simulink model "test_ntc"  (R2018a)
settings: Solver=ode1  StartTime=0.0  StopTime=8  FixedStep=1e-3  RelTol=1e-3
undefined symbols (not defined in the file): ntc10k
libraries: fl_lib x19, nesl_utility x6, elec_lib x2, simulink x2
settings Model: Creator=ChLan  LastModifiedBy=ChLan
settings SimscapeCC: SimscapeNormalizeSystem=off  SimscapeLogType=all  SimscapeLogToSDI=on

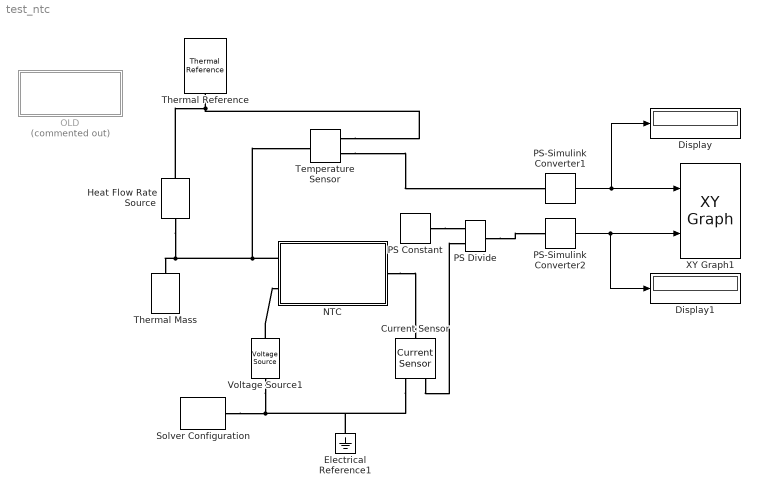
== system test_ntc ==
  Current Sensor : fl_lib/Electrical/Electrical Sensors/Current Sensor
  Display : Display
  Display1 : Display
  Electrical Reference1 : fl_lib/Electrical/Electrical Elements/Electrical Reference
  Heat Flow Rate Source : fl_lib/Thermal/Thermal Sources/Heat Flow Rate Source  heat_flow=10 W
      settings: SourceProductName=Simscape  SourceProductBaseCode=SS
  NTC : Subsystem  mask{res_table=ntc10k}
      mask prompts: res_table "T-R Table"
  OLD : Subsystem  Commented=on
  PS Constant : fl_lib/Physical Signals/Sources/PS Constant  constant=1000
  PS Divide : fl_lib/Physical Signals/Functions/PS Divide
      settings: SourceProductName=Simscape  SourceProductBaseCode=SS
  PS-Simulink Converter1 : nesl_utility/PS-Simulink Converter  PhysicalDomain=network_engine_domain  SubClassName=ps_output  LeftPortType=input  RightPortType=output  PseudoPeriodic=off  Frequencies=[]  Unit=degC  AffineConversion=on
  PS-Simulink Converter2 : nesl_utility/PS-Simulink Converter  PhysicalDomain=network_engine_domain  SubClassName=ps_output  LeftPortType=input  RightPortType=output  PseudoPeriodic=off  Frequencies=[]  Unit=1  AffineConversion=off
  Solver Configuration : nesl_utility/Solver Configuration  PhysicalDomain=network_engine_domain  SubClassName=solver  LeftPortType=input  RightPortType=generic  Tones=[]  Harmonics=[]  SimulateNoise=off  Profile=off  UseLocalSampling=off  EnableSwitchedLinearOptims=on  FrequencyDomain=off  UseCCode=off  RelTol=0.001  AbsTol=1e-06  MinStep=1e-09  ToWorkspace=off  RevertToSquareIcSolve=off  NumHomotopyIterations=100  PhasorMode=off  PhasorModeNumHarmonics=1  DoDC=off  ResidualTolerance=1e-09  UseLocalSolver=off  LocalSolverChoice=NE_BACKWARD_EULER_ADVANCER  LocalSolverSampleTime=0.001  DoFixedCost=off  MaxNonlinIter=3  MaxModeIter=2  LinearAlgebra=Sparse  EquationFormulation=NE_TIME_EF  DelaysMemoryBudget=1024  AutomaticFiltering=on  FilteringTimeConstant=0.001
  Temperature Sensor : fl_lib/Thermal/Thermal Sensors/Temperature Sensor
  Thermal Mass : fl_lib/Thermal/Thermal Elements/Thermal Mass  mass=1 kg  sp_heat=1 J/kg/K  T_specify=on  T_priority=High  T=298 K  T_nominal_specify=off  T_nominal_unit=K  T_nominal_value=1  Q_specify=off  Q_priority=None  Q=0 W  Q_nominal_specify=off  Q_nominal_unit=W  Q_nominal_value=1
  Thermal Reference : fl_lib/Thermal/Thermal Elements/Thermal Reference
  Voltage Source1 : elec_lib/Sources/Voltage Source  dc_voltage=1000 V  ac_voltage=0 V  ac_shift=0 rad  ac_frequency=60 Hz  noise_mode=0  PSD=0 V^2/Hz  repeatability=1  auto_seed=793780051  user_seed=0  sample_time=1e-3 s  i_specify=off  i_priority=None  i=0 A  i_nominal_specify=off  i_nominal_unit=A  i_nominal_value=1  v_specify=off  v_priority=None  v=0 V  v_nominal_specify=off  v_nominal_unit=V  v_nominal_value=1
      settings: SourceProductName=Simscape Electronics  SourceProductBaseCode=SN
  XY Graph1 : simulink/Sinks/XY Graph  xmin=20  xmax=100  ymin=100  ymax=10000  st=-1
  wires:
  PS-Simulink Converter1/1 -> XY Graph1/1, Display/1
  PS-Simulink Converter2/1 -> XY Graph1/2, Display1/1
  connections:
  Voltage Source1/RConn1 -- Current Sensor/RConn2 -- Electrical Reference1/LConn1 -- Solver Configuration/RConn1
  NTC/LConn1 -- Temperature Sensor/LConn1 -- Heat Flow Rate Source/LConn1 -- Thermal Mass/LConn1
  Voltage Source1/LConn1 -- NTC/LConn2
  Temperature Sensor/RConn1 -- Heat Flow Rate Source/RConn1 -- Thermal Reference/LConn1
  Temperature Sensor/RConn2 -- PS-Simulink Converter1/LConn1
  NTC/RConn1 -- Current Sensor/LConn1
  Current Sensor/RConn1 -- PS Divide/LConn2
  PS Constant/RConn1 -- PS Divide/LConn1
  PS Divide/RConn1 -- PS-Simulink Converter2/LConn1

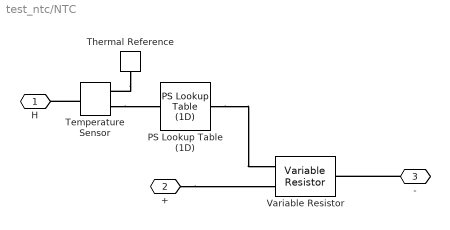
== system test_ntc/NTC ==
  PS Lookup Table (1D) : fl_lib/Physical Signals/Lookup Tables/PS Lookup Table (1D)  x=res_table(:,1) + 273.2  f=res_table(:,2)  interp_method=simscape.enum.interpolation.linear  extrap_method=simscape.enum.extrapolation.linear
      settings: SourceProductName=Simscape  SourceProductBaseCode=SS
  Temperature Sensor : fl_lib/Thermal/Thermal Sensors/Temperature Sensor
  Thermal Reference : fl_lib/Thermal/Thermal Elements/Thermal Reference
  Variable Resistor : fl_lib/Electrical/Electrical Elements/Variable Resistor  Rmin=0 Ohm  i_specify=off  i_priority=None  i=0 A  i_nominal_specify=off  i_nominal_unit=A  i_nominal_value=1  v_specify=off  v_priority=None  v=0 V  v_nominal_specify=off  v_nominal_unit=V  v_nominal_value=1
  H : PMIOPort  Side=Left
  + : PMIOPort  Port=2  Side=Left
  - : PMIOPort  Port=3  Side=Right
  connections:
  PS Lookup Table (1D)/RConn1 -- Variable Resistor/LConn1
  Temperature Sensor/RConn2 -- PS Lookup Table (1D)/LConn1
  +/RConn1 -- Variable Resistor/LConn2
  Temperature Sensor/LConn1 -- H/RConn1
  Thermal Reference/LConn1 -- Temperature Sensor/RConn1
  -/RConn1 -- Variable Resistor/RConn1

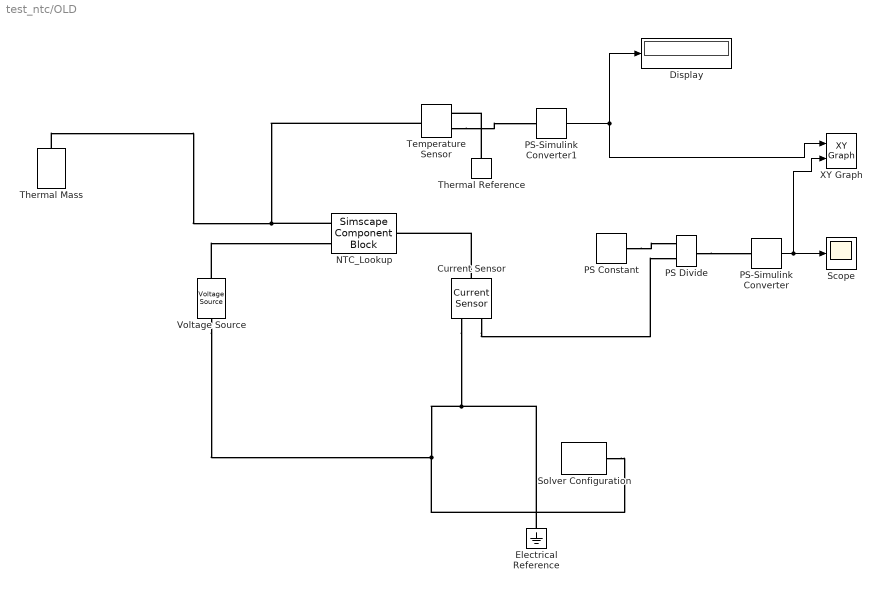
== system test_ntc/OLD ==
  Current Sensor : fl_lib/Electrical/Electrical Sensors/Current Sensor
  Display : Display
  Electrical Reference : fl_lib/Electrical/Electrical Elements/Electrical Reference
  NTC_Lookup : SimscapeComponentBlock  SourceFile=ntc_lookup  ComponentPath=ntc_lookup  ComponentVariants=ntc_lookup  ComponentVariantNames=ntc_lookup  ClassName=ntc_lookup  SchemaVersion=1  C=10 J/K  res_t=ntc10k(:,1) degC  res_r=ntc10k(:,2) Ohm  T_specify=on  T_priority=High  T=298 K  T_nominal_specify=off  T_nominal_unit=K  T_nominal_value=1
      settings: CopyFcn=simscape.engine.sli.internal.componentblockcallback(gcbh,'COPY')  PreCopyFcn=simscape.engine.sli.internal.componentblockcallback(gcbh,'PRECOPY')  PreDeleteFcn=simscape.engine.sli.internal.componentblockcallback(gcbh,'PREDELETE')  LogSimulationData=on
      mask Type: NTC-Resistor with Lookup-Table
  PS Constant : fl_lib/Physical Signals/Sources/PS Constant  constant=1000
  PS Divide : fl_lib/Physical Signals/Functions/PS Divide
      settings: SourceProductName=Simscape  SourceProductBaseCode=SS
  PS-Simulink Converter : nesl_utility/PS-Simulink Converter  PhysicalDomain=network_engine_domain  SubClassName=ps_output  LeftPortType=input  RightPortType=output  PseudoPeriodic=off  Frequencies=[]  Unit=1  AffineConversion=off
  PS-Simulink Converter1 : nesl_utility/PS-Simulink Converter  PhysicalDomain=network_engine_domain  SubClassName=ps_output  LeftPortType=input  RightPortType=output  PseudoPeriodic=off  Frequencies=[]  Unit=degC  AffineConversion=on
  Scope : Scope
  Solver Configuration : nesl_utility/Solver Configuration  PhysicalDomain=network_engine_domain  SubClassName=solver  LeftPortType=input  RightPortType=generic  Tones=[]  Harmonics=[]  SimulateNoise=off  Profile=off  UseLocalSampling=off  EnableSwitchedLinearOptims=on  FrequencyDomain=off  UseCCode=off  RelTol=0.001  AbsTol=1e-06  MinStep=1e-09  ToWorkspace=off  RevertToSquareIcSolve=off  NumHomotopyIterations=100  PhasorMode=off  PhasorModeNumHarmonics=1  DoDC=off  ResidualTolerance=1e-09  UseLocalSolver=off  LocalSolverChoice=NE_BACKWARD_EULER_ADVANCER  LocalSolverSampleTime=0.001  DoFixedCost=off  MaxNonlinIter=3  MaxModeIter=2  LinearAlgebra=Sparse  EquationFormulation=NE_TIME_EF  DelaysMemoryBudget=1024  AutomaticFiltering=on  FilteringTimeConstant=0.001
  Temperature Sensor : fl_lib/Thermal/Thermal Sensors/Temperature Sensor
  Thermal Mass : fl_lib/Thermal/Thermal Elements/Thermal Mass  mass=100 g  sp_heat=447 J/kg/K  T_specify=off  T_priority=High  T=300 K  T_nominal_specify=off  T_nominal_unit=K  T_nominal_value=1  Q_specify=off  Q_priority=None  Q=0 W  Q_nominal_specify=off  Q_nominal_unit=W  Q_nominal_value=1
  Thermal Reference : fl_lib/Thermal/Thermal Elements/Thermal Reference
  Voltage Source : elec_lib/Sources/Voltage Source  dc_voltage=1000 V  ac_voltage=0 V  ac_shift=0 rad  ac_frequency=60 Hz  noise_mode=0  PSD=0 V^2/Hz  repeatability=1  auto_seed=2680317669  user_seed=0  sample_time=1e-3 s  i_specify=off  i_priority=None  i=0 A  i_nominal_specify=off  i_nominal_unit=A  i_nominal_value=1  v_specify=off  v_priority=None  v=0 V  v_nominal_specify=off  v_nominal_unit=V  v_nominal_value=1
      settings: SourceProductName=Simscape Electronics  SourceProductBaseCode=SN
  XY Graph : simulink/Sinks/XY Graph  xmin=20  xmax=100  ymin=100  ymax=10000  st=-1
  wires:
  PS-Simulink Converter1/1 -> XY Graph/1, Display/1
  PS-Simulink Converter/1 -> XY Graph/2, Scope/1
  connections:
  Electrical Reference/LConn1 -- Voltage Source/RConn1 -- Solver Configuration/RConn1 -- Current Sensor/RConn2
  Temperature Sensor/RConn2 -- PS-Simulink Converter1/LConn1
  Temperature Sensor/LConn1 -- Thermal Mass/LConn1 -- NTC_Lookup/LConn1
  Thermal Reference/LConn1 -- Temperature Sensor/RConn1
  Current Sensor/LConn1 -- NTC_Lookup/RConn1
  PS Divide/RConn1 -- PS-Simulink Converter/LConn1
  Voltage Source/LConn1 -- NTC_Lookup/LConn2
  PS Constant/RConn1 -- PS Divide/LConn1
  Current Sensor/RConn1 -- PS Divide/LConn2
